simulink model "model5"  (R2022a)
settings: Solver=FixedStepAuto  StartTime=0.0  StopTime=100  FixedStep=0.001  RelTol=1e-3
undefined symbols (not defined in the file): A, A2, B, B2, C, C2, D, D2, K1, K2, w0, x0
settings Model: Creator=Дети  LastModifiedBy=Rynsi
settings ModelReferenceCC: EnableRefExpFcnMdlSchedulingChecks=off
settings RTWCC: Description=Generic Real-Time Target

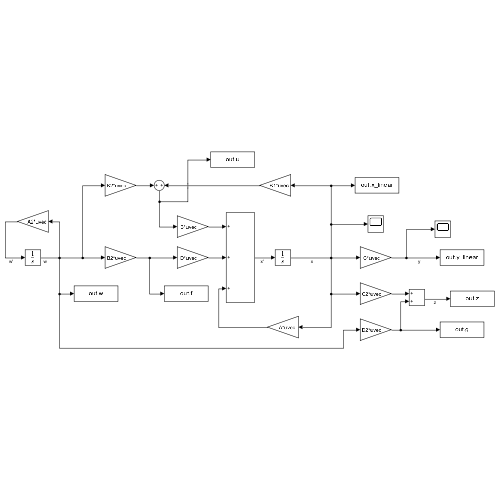
[thumbnail: Simulink's stored preview of the top-level diagram]
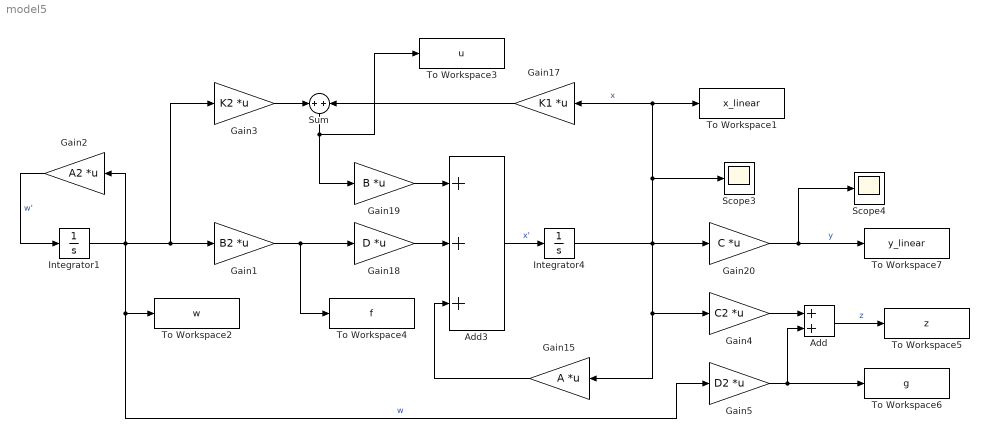
== system model5 ==
  Add : Sum
  Add3 : Sum  Inputs=+++
  Gain1 : Gain  Gain=B2  Multiplication=Matrix(K*u) (u vector)
  Gain15 : Gain  Gain=A  Multiplication=Matrix(K*u) (u vector)
  Gain17 : Gain  Gain=K1  Multiplication=Matrix(K*u) (u vector)
  Gain18 : Gain  Gain=D  Multiplication=Matrix(K*u) (u vector)
  Gain19 : Gain  Gain=B  Multiplication=Matrix(K*u) (u vector)
  Gain2 : Gain  Gain=A2  Multiplication=Matrix(K*u) (u vector)
  Gain20 : Gain  Gain=C  Multiplication=Matrix(K*u) (u vector)
  Gain3 : Gain  Gain=K2  Multiplication=Matrix(K*u) (u vector)
  Gain4 : Gain  Gain=C2  Multiplication=Matrix(K*u) (u vector)
  Gain5 : Gain  Gain=D2  Multiplication=Matrix(K*u) (u vector)
  Integrator1 : Integrator  InitialCondition=w0
  Integrator4 : Integrator  InitialCondition=x0
  Scope3 : Scope
  Scope4 : Scope
  Sum : Sum  Inputs=+|+
  To Workspace1 : ToWorkspace  VariableName=x_linear  SaveFormat=Timeseries  SampleTime=-1
  To Workspace2 : ToWorkspace  VariableName=w  SaveFormat=Timeseries  SampleTime=-1
  To Workspace3 : ToWorkspace  VariableName=u  SaveFormat=Timeseries  SampleTime=-1
  To Workspace4 : ToWorkspace  VariableName=f  SaveFormat=Timeseries  SampleTime=-1
  To Workspace5 : ToWorkspace  VariableName=z  SaveFormat=Timeseries  SampleTime=-1
  To Workspace6 : ToWorkspace  VariableName=g  SaveFormat=Timeseries  SampleTime=-1
  To Workspace7 : ToWorkspace  VariableName=y_linear  SaveFormat=Timeseries  SampleTime=-1
  wires:
  Add3/1 -> Integrator4/1  "x'"
  Integrator4/1 -> Gain17/1, To Workspace1/1, Scope3/1, Gain20/1, Gain4/1, Gain15/1  "x"
  Gain15/1 -> Add3/3
  Gain18/1 -> Add3/2
  Gain20/1 -> Scope4/1, To Workspace7/1  "y"
  Gain2/1 -> Integrator1/1  "w'"
  Integrator1/1 -> Gain5/1, To Workspace2/1, Gain3/1, Gain1/1, Gain2/1  "w"
  Gain19/1 -> Add3/1
  Sum/1 -> To Workspace3/1, Gain19/1
  Gain17/1 -> Sum/2
  Gain3/1 -> Sum/1
  Gain1/1 -> To Workspace4/1, Gain18/1
  Add/1 -> To Workspace5/1  "z"
  Gain4/1 -> Add/1
  Gain5/1 -> To Workspace6/1, Add/2
